simulink model "case2"  (R2024b)
settings: Solver=FixedStepAuto  StartTime=0  StopTime=1  FixedStep=1e-7  RelTol=1e-3
values from neighbouring files (symbols this model uses):
  SG_D_1_D = 0.01056    [IEEE9_case_parameters.m]    (also in case1_parameters.m; case2_parameters.m; case3_parameters.m; case4_parameters.m)
  SG_D_1_EnableSaturation = 0    [IEEE9_case_parameters.m]    (also in case1_parameters.m; case2_parameters.m; case3_parameters.m; case4_parameters.m)
  SG_D_1_f0 = 60    [IEEE9_case_parameters.m]    (also in case1_parameters.m; case2_parameters.m; case3_parameters.m; case4_parameters.m)
  SG_D_1_H = 7.5    [IEEE9_case_parameters.m]    (also in case1_parameters.m; case2_parameters.m; case3_parameters.m; case4_parameters.m)
  SG_D_1_K_A = 20    [IEEE9_case_parameters.m]    (also in case1_parameters.m; case2_parameters.m; case3_parameters.m; case4_parameters.m)
  SG_D_1_K_E = 1.000000e+1    (= 10)    [IEEE9_case_parameters.m]    (also in case1_parameters.m; case2_parameters.m; case3_parameters.m; case4_parameters.m)
  SG_D_1_K_F = 2.363    [IEEE9_case_parameters.m]    (also in case1_parameters.m; case2_parameters.m; case3_parameters.m; case4_parameters.m)
  SG_D_1_K_s = 0.5    [IEEE9_case_parameters.m]    (also in case1_parameters.m = 5; case2_parameters.m = 5; case3_parameters.m = 5; case4_parameters.m = 5)
  SG_D_1_R_a = 0.001088    [IEEE9_case_parameters.m]    (also in case1_parameters.m; case2_parameters.m; case3_parameters.m; case4_parameters.m)
  SG_D_1_S_A = 1    [IEEE9_case_parameters.m]    (also in case1_parameters.m; case2_parameters.m; case3_parameters.m; case4_parameters.m)
  SG_D_1_S_B = 0.103    [IEEE9_case_parameters.m]    (also in case1_parameters.m; case2_parameters.m; case3_parameters.m; case4_parameters.m)
  SG_D_1_S_N = 10.659857    [IEEE9_case_parameters.m]    (also in case1_parameters.m; case2_parameters.m; case3_parameters.m; case4_parameters.m)
  SG_D_1_SpeedPara = 200    [IEEE9_case_parameters.m]    (also in case1_parameters.m; case2_parameters.m; case3_parameters.m; case4_parameters.m)
  SG_D_1_T_0 = 0.720173    [IEEE9_case_parameters.m]    (also in case1_parameters.m = 0.755522; case2_parameters.m = 0.808931; case3_parameters.m = 0.869402; case4_parameters.m = 0.729316)
  SG_D_1_T_1 = 0.3    [IEEE9_case_parameters.m]    (also in case1_parameters.m; case2_parameters.m; case3_parameters.m; case4_parameters.m)
  SG_D_1_T_2 = 0.05    [IEEE9_case_parameters.m]    (also in case1_parameters.m; case2_parameters.m; case3_parameters.m; case4_parameters.m)
  SG_D_1_T_3 = 0.02    [IEEE9_case_parameters.m]    (also in case1_parameters.m; case2_parameters.m; case3_parameters.m; case4_parameters.m)
  SG_D_1_T_4 = 0.005    [IEEE9_case_parameters.m]    (also in case1_parameters.m; case2_parameters.m; case3_parameters.m; case4_parameters.m)
  SG_D_1_T_A = 0.02    [IEEE9_case_parameters.m]    (also in case1_parameters.m; case2_parameters.m; case3_parameters.m; case4_parameters.m)
  SG_D_1_T_dd = 8.000000e+0    (= 8)    [IEEE9_case_parameters.m]    (also in case1_parameters.m; case2_parameters.m; case3_parameters.m; case4_parameters.m)
  SG_D_1_T_ddd = 0.04    [IEEE9_case_parameters.m]    (also in case1_parameters.m; case2_parameters.m; case3_parameters.m; case4_parameters.m)
  SG_D_1_T_E = 0.314    [IEEE9_case_parameters.m]    (also in case1_parameters.m; case2_parameters.m; case3_parameters.m; case4_parameters.m)
  SG_D_1_T_F = 0.35    [IEEE9_case_parameters.m]    (also in case1_parameters.m; case2_parameters.m; case3_parameters.m; case4_parameters.m)
  SG_D_1_T_qd = 0.8    [IEEE9_case_parameters.m]    (also in case1_parameters.m; case2_parameters.m; case3_parameters.m; case4_parameters.m)
  SG_D_1_T_qdd = 0.02    [IEEE9_case_parameters.m]    (also in case1_parameters.m; case2_parameters.m; case3_parameters.m; case4_parameters.m)
  SG_D_1_T_speed = 0.1    [IEEE9_case_parameters.m]    (also in case1_parameters.m = 200; case2_parameters.m = 200; case3_parameters.m = 200; case4_parameters.m = 200)
  SG_D_1_T_w = 0.5    [IEEE9_case_parameters.m]    (also in case1_parameters.m; case2_parameters.m; case3_parameters.m; case4_parameters.m)
  SG_D_1_V_ref = 1.990276    [IEEE9_case_parameters.m]    (also in case1_parameters.m = 2.042296; case2_parameters.m = 2.051388; case3_parameters.m = 2.089584; case4_parameters.m = 2.01845)
  SG_D_1_w_ref = 376.991118    [IEEE9_case_parameters.m]    (also in case1_parameters.m; case2_parameters.m; case3_parameters.m; case4_parameters.m)
  SG_D_1_wb = 6.000000e+1    (= 60)    [IEEE9_case_parameters.m]    (also in case1_parameters.m; case2_parameters.m; case3_parameters.m; case4_parameters.m)
  SG_D_1_x_d = 1.9    [IEEE9_case_parameters.m]    (also in case1_parameters.m; case2_parameters.m; case3_parameters.m; case4_parameters.m)
  SG_D_1_x_dd = 0.302    [IEEE9_case_parameters.m]    (also in case1_parameters.m; case2_parameters.m; case3_parameters.m; case4_parameters.m)
  SG_D_1_x_ddd = 0.204    [IEEE9_case_parameters.m]    (also in case1_parameters.m; case2_parameters.m; case3_parameters.m; case4_parameters.m)
  SG_D_1_x_l = 0.05    [IEEE9_case_parameters.m]    (also in case1_parameters.m; case2_parameters.m; case3_parameters.m; case4_parameters.m)
  SG_D_1_x_q = 1.3    [IEEE9_case_parameters.m]    (also in case1_parameters.m; case2_parameters.m; case3_parameters.m; case4_parameters.m)
  SG_D_1_x_qd = 0.5    [IEEE9_case_parameters.m]    (also in case1_parameters.m; case2_parameters.m; case3_parameters.m; case4_parameters.m)
  SG_D_1_x_qdd = 0.3    [IEEE9_case_parameters.m]    (also in case1_parameters.m; case2_parameters.m; case3_parameters.m; case4_parameters.m)
  SG_D_2_D = 0.02    [IEEE9_case_parameters.m]    (also in case1_parameters.m; case2_parameters.m; case3_parameters.m; case4_parameters.m)
  SG_D_2_EnableSaturation = 0    [IEEE9_case_parameters.m]    (also in case1_parameters.m; case2_parameters.m; case3_parameters.m; case4_parameters.m)
  SG_D_2_f0 = 60    [IEEE9_case_parameters.m]    (also in case1_parameters.m; case2_parameters.m; case3_parameters.m; case4_parameters.m)
  SG_D_2_H = 8.000000e+0    (= 8)    [IEEE9_case_parameters.m]    (also in case1_parameters.m; case2_parameters.m; case3_parameters.m; case4_parameters.m)
  SG_D_2_K_A = 20    [IEEE9_case_parameters.m]    (also in case1_parameters.m; case2_parameters.m; case3_parameters.m; case4_parameters.m)
  SG_D_2_K_E = 1.000000e+1    (= 10)    [IEEE9_case_parameters.m]    (also in case1_parameters.m; case2_parameters.m; case3_parameters.m; case4_parameters.m)
  SG_D_2_K_F = 2.363    [IEEE9_case_parameters.m]    (also in case1_parameters.m; case2_parameters.m; case3_parameters.m; case4_parameters.m)
  SG_D_2_K_s = 0.5    [IEEE9_case_parameters.m]    (also in case1_parameters.m = 4; case2_parameters.m = 4; case3_parameters.m = 4; case4_parameters.m = 4)
  SG_D_2_R_a = 0.001088    [IEEE9_case_parameters.m]    (also in case1_parameters.m; case2_parameters.m; case3_parameters.m; case4_parameters.m)
  SG_D_2_S_A = 1    [IEEE9_case_parameters.m]    (also in case1_parameters.m; case2_parameters.m; case3_parameters.m; case4_parameters.m)
  SG_D_2_S_B = 0.103    [IEEE9_case_parameters.m]    (also in case1_parameters.m; case2_parameters.m; case3_parameters.m; case4_parameters.m)
  SG_D_2_S_N = 10.659857    [IEEE9_case_parameters.m]    (also in case1_parameters.m; case2_parameters.m; case3_parameters.m; case4_parameters.m)
  SG_D_2_SpeedPara = 200    [IEEE9_case_parameters.m]    (also in case1_parameters.m; case2_parameters.m; case3_parameters.m; case4_parameters.m)
  SG_D_2_T_0 = 1.632913    [IEEE9_case_parameters.m]    (also in case1_parameters.m = 1.632925; case2_parameters.m = 1.632915; case3_parameters.m = 1.632914; case4_parameters.m = 1.632927)
  SG_D_2_T_1 = 0.2    [IEEE9_case_parameters.m]    (also in case1_parameters.m; case2_parameters.m; case3_parameters.m; case4_parameters.m)
  SG_D_2_T_2 = 0.05    [IEEE9_case_parameters.m]    (also in case1_parameters.m; case2_parameters.m; case3_parameters.m; case4_parameters.m)
  SG_D_2_T_3 = 0.02    [IEEE9_case_parameters.m]    (also in case1_parameters.m; case2_parameters.m; case3_parameters.m; case4_parameters.m)
  SG_D_2_T_4 = 0.005    [IEEE9_case_parameters.m]    (also in case1_parameters.m; case2_parameters.m; case3_parameters.m; case4_parameters.m)
  SG_D_2_T_A = 0.02    [IEEE9_case_parameters.m]    (also in case1_parameters.m; case2_parameters.m; case3_parameters.m; case4_parameters.m)
  SG_D_2_T_dd = 7.9    [IEEE9_case_parameters.m]    (also in case1_parameters.m; case2_parameters.m; case3_parameters.m; case4_parameters.m)
  SG_D_2_T_ddd = 0.04    [IEEE9_case_parameters.m]    (also in case1_parameters.m; case2_parameters.m; case3_parameters.m; case4_parameters.m)
  SG_D_2_T_E = 0.314    [IEEE9_case_parameters.m]    (also in case1_parameters.m; case2_parameters.m; case3_parameters.m; case4_parameters.m)
  SG_D_2_T_F = 0.35    [IEEE9_case_parameters.m]    (also in case1_parameters.m; case2_parameters.m; case3_parameters.m; case4_parameters.m)
  SG_D_2_T_qd = 0.8    [IEEE9_case_parameters.m]    (also in case1_parameters.m; case2_parameters.m; case3_parameters.m; case4_parameters.m)
  SG_D_2_T_qdd = 0.015    [IEEE9_case_parameters.m]    (also in case1_parameters.m; case2_parameters.m; case3_parameters.m; case4_parameters.m)
  SG_D_2_T_speed = 0.1    [IEEE9_case_parameters.m]    (also in case1_parameters.m = 150; case2_parameters.m = 150; case3_parameters.m = 150; case4_parameters.m = 150)
  SG_D_2_T_w = 0.35    [IEEE9_case_parameters.m]    (also in case1_parameters.m; case2_parameters.m; case3_parameters.m; case4_parameters.m)
  SG_D_2_V_ref = 2.58547    [IEEE9_case_parameters.m]    (also in case1_parameters.m = 2.597896; case2_parameters.m = 2.587136; case3_parameters.m = 2.586042; case4_parameters.m = 2.599679)
  SG_D_2_w_ref = 376.991118    [IEEE9_case_parameters.m]    (also in case1_parameters.m; case2_parameters.m; case3_parameters.m; case4_parameters.m)
  SG_D_2_wb = 6.000000e+1    (= 60)    [IEEE9_case_parameters.m]    (also in case1_parameters.m; case2_parameters.m; case3_parameters.m; case4_parameters.m)
  SG_D_2_x_d = 1.8    [IEEE9_case_parameters.m]    (also in case1_parameters.m; case2_parameters.m; case3_parameters.m; case4_parameters.m)
  SG_D_2_x_dd = 0.302    [IEEE9_case_parameters.m]    (also in case1_parameters.m; case2_parameters.m; case3_parameters.m; case4_parameters.m)
  SG_D_2_x_ddd = 0.204    [IEEE9_case_parameters.m]    (also in case1_parameters.m; case2_parameters.m; case3_parameters.m; case4_parameters.m)
  SG_D_2_x_l = 0.05    [IEEE9_case_parameters.m]    (also in case1_parameters.m; case2_parameters.m; case3_parameters.m; case4_parameters.m)
  SG_D_2_x_q = 1.25    [IEEE9_case_parameters.m]    (also in case1_parameters.m; case2_parameters.m; case3_parameters.m; case4_parameters.m)
  SG_D_2_x_qd = 0.5    [IEEE9_case_parameters.m]    (also in case1_parameters.m; case2_parameters.m; case3_parameters.m; case4_parameters.m)
  SG_D_2_x_qdd = 0.3    [IEEE9_case_parameters.m]    (also in case1_parameters.m; case2_parameters.m; case3_parameters.m; case4_parameters.m)
  SG_D_3_D = 0.02    [IEEE9_case_parameters.m]    (also in case1_parameters.m; case2_parameters.m; case3_parameters.m; case4_parameters.m)
  SG_D_3_EnableSaturation = 0    [IEEE9_case_parameters.m]    (also in case1_parameters.m; case2_parameters.m; case3_parameters.m; case4_parameters.m)
  SG_D_3_f0 = 60    [IEEE9_case_parameters.m]    (also in case1_parameters.m; case2_parameters.m; case3_parameters.m; case4_parameters.m)
  SG_D_3_H = 7.7    [IEEE9_case_parameters.m]    (also in case1_parameters.m; case2_parameters.m; case3_parameters.m; case4_parameters.m)
  SG_D_3_K_A = 20    [IEEE9_case_parameters.m]    (also in case1_parameters.m; case2_parameters.m; case3_parameters.m; case4_parameters.m)
  SG_D_3_K_E = 1.000000e+1    (= 10)    [IEEE9_case_parameters.m]    (also in case1_parameters.m; case2_parameters.m; case3_parameters.m; case4_parameters.m)
  SG_D_3_K_F = 2.363    [IEEE9_case_parameters.m]    (also in case1_parameters.m; case2_parameters.m; case3_parameters.m; case4_parameters.m)
  SG_D_3_K_s = 0.2    [IEEE9_case_parameters.m]    (also in case1_parameters.m = 2; case2_parameters.m = 2; case3_parameters.m = 2; case4_parameters.m = 2)
  SG_D_3_R_a = 0.001088    [IEEE9_case_parameters.m]    (also in case1_parameters.m; case2_parameters.m; case3_parameters.m; case4_parameters.m)
  SG_D_3_S_A = 1    [IEEE9_case_parameters.m]    (also in case1_parameters.m; case2_parameters.m; case3_parameters.m; case4_parameters.m)
  SG_D_3_S_B = 0.103    [IEEE9_case_parameters.m]    (also in case1_parameters.m; case2_parameters.m; case3_parameters.m; case4_parameters.m)
  SG_D_3_S_N = 10.659857    [IEEE9_case_parameters.m]    (also in case1_parameters.m; case2_parameters.m; case3_parameters.m; case4_parameters.m)
  SG_D_3_SpeedPara = 200    [IEEE9_case_parameters.m]    (also in case1_parameters.m; case2_parameters.m; case3_parameters.m; case4_parameters.m)
  SG_D_3_T_0 = 0.850788    [IEEE9_case_parameters.m]    (also in case1_parameters.m = 0.850786; case2_parameters.m = 0.850787; case3_parameters.m; case4_parameters.m = 0.850786)
  SG_D_3_T_1 = 0.2    [IEEE9_case_parameters.m]    (also in case1_parameters.m; case2_parameters.m; case3_parameters.m; case4_parameters.m)
  SG_D_3_T_2 = 0.05    [IEEE9_case_parameters.m]    (also in case1_parameters.m; case2_parameters.m; case3_parameters.m; case4_parameters.m)
  SG_D_3_T_3 = 0.02    [IEEE9_case_parameters.m]    (also in case1_parameters.m; case2_parameters.m; case3_parameters.m; case4_parameters.m)
  SG_D_3_T_4 = 0.005    [IEEE9_case_parameters.m]    (also in case1_parameters.m; case2_parameters.m; case3_parameters.m; case4_parameters.m)
  SG_D_3_T_A = 0.02    [IEEE9_case_parameters.m]    (also in case1_parameters.m; case2_parameters.m; case3_parameters.m; case4_parameters.m)
  SG_D_3_T_dd = 8.1    [IEEE9_case_parameters.m]    (also in case1_parameters.m; case2_parameters.m; case3_parameters.m; case4_parameters.m)
  SG_D_3_T_ddd = 0.04    [IEEE9_case_parameters.m]    (also in case1_parameters.m; case2_parameters.m; case3_parameters.m; case4_parameters.m)
  SG_D_3_T_E = 0.314    [IEEE9_case_parameters.m]    (also in case1_parameters.m; case2_parameters.m; case3_parameters.m; case4_parameters.m)
  SG_D_3_T_F = 0.35    [IEEE9_case_parameters.m]    (also in case1_parameters.m; case2_parameters.m; case3_parameters.m; case4_parameters.m)
  SG_D_3_T_qd = 0.8    [IEEE9_case_parameters.m]    (also in case1_parameters.m; case2_parameters.m; case3_parameters.m; case4_parameters.m)
  SG_D_3_T_qdd = 0.015    [IEEE9_case_parameters.m]    (also in case1_parameters.m; case2_parameters.m; case3_parameters.m; case4_parameters.m)
  SG_D_3_T_speed = 0.1    [IEEE9_case_parameters.m]    (also in case1_parameters.m = 180; case2_parameters.m = 180; case3_parameters.m = 180; case4_parameters.m = 180)
  SG_D_3_T_w = 0.4    [IEEE9_case_parameters.m]    (also in case1_parameters.m; case2_parameters.m; case3_parameters.m; case4_parameters.m)
  SG_D_3_V_ref = 1.892727    [IEEE9_case_parameters.m]    (also in case1_parameters.m = 1.906439; case2_parameters.m = 1.895535; case3_parameters.m = 1.892105; case4_parameters.m = 1.906598)
  SG_D_3_w_ref = 376.991118    [IEEE9_case_parameters.m]    (also in case1_parameters.m; case2_parameters.m; case3_parameters.m; case4_parameters.m)
  SG_D_3_wb = 6.000000e+1    (= 60)    [IEEE9_case_parameters.m]    (also in case1_parameters.m; case2_parameters.m; case3_parameters.m; case4_parameters.m)
  SG_D_3_x_d = 1.85    [IEEE9_case_parameters.m]    (also in case1_parameters.m; case2_parameters.m; case3_parameters.m; case4_parameters.m)
  SG_D_3_x_dd = 0.302    [IEEE9_case_parameters.m]    (also in case1_parameters.m; case2_parameters.m; case3_parameters.m; case4_parameters.m)
  SG_D_3_x_ddd = 0.204    [IEEE9_case_parameters.m]    (also in case1_parameters.m; case2_parameters.m; case3_parameters.m; case4_parameters.m)
  SG_D_3_x_l = 0.05    [IEEE9_case_parameters.m]    (also in case1_parameters.m; case2_parameters.m; case3_parameters.m; case4_parameters.m)
  SG_D_3_x_q = 1.2    [IEEE9_case_parameters.m]    (also in case1_parameters.m; case2_parameters.m; case3_parameters.m; case4_parameters.m)
  SG_D_3_x_qd = 0.5    [IEEE9_case_parameters.m]    (also in case1_parameters.m; case2_parameters.m; case3_parameters.m; case4_parameters.m)
  SG_D_3_x_qdd = 0.3    [IEEE9_case_parameters.m]    (also in case1_parameters.m; case2_parameters.m; case3_parameters.m; case4_parameters.m)
(part 8 of 12)

== system case2/SG_D_2/d_psi_d_SG_D_2_block ==
  note: d_psi_d_SG_D_2 in case2
      | $2\,\pi \,f_{0}\,\left(v_{d,\mathrm{SG},D,2}\,\sin\left(\theta _{\mathrm{SG},D,2}\right)-v_{q,\mathrm{SG},D,2}\,\cos\left(\theta _{\mathrm{SG},D,2}\right)+\frac{R_{a}\,\left(\frac{\psi _{\mathrm{1d},\mathrm{SG},D,2}\,\left(x_{\mathrm{dd}}-x_{\mathrm{ddd}}\right)}{x_{\mathrm{dd}}-x_{l}}-\psi _{d,\mathrm{SG},D,2}+\frac{\psi _{\mathrm{fd},\mathrm{SG},D,2}\,\left(x_{\mathrm{ddd}}-x_{l}\right)}{x_{\mathrm{dd}}-x_{l}}\right)}{x_{\mathrm{ddd}}}+\frac{\psi _{q,\mathrm{SG},D,2}\,w_{\mathrm{SG},D,2}}{2\,f_{0}\,\pi }\right)$
      | Automatically generated on 2025-10-31 18:54:12 .
  State_psi_1d_SG_D_2_3fdee : Inport
  State_psi_d_SG_D_2_d60ed : Inport  Port=2
  State_psi_fd_SG_D_2_19126 : Inport  Port=3
  Input_v_d_SG_D_2_3ae72 : Inport  Port=4
  State_theta_SG_D_2_01400 : Inport  Port=5
  Input_v_q_SG_D_2_cabf7 : Inport  Port=6
  State_theta_SG_D_2_a0973 : Inport  Port=7
  State_psi_q_SG_D_2_fe7e7 : Inport  Port=8
  State_w_SG_D_2_e892d : Inport  Port=9
  Add_2c66e : Sum
  Add_408a3 : Sum
  Constant_-1_07947 : Constant  Value=-1
  Constant_-2.0_4d0c8 : Constant  Value=-2.0
  Constant_2.0_2af4c : Constant  Value=2.0
  Constant_R_a_dbd06 : Constant  Value=R_a
  Constant_f0_83e57 : Constant  Value=f0
  Constant_f0_9e5d9 : Constant  Value=f0
  Constant_pi_c86ee : Constant  Value=pi
  Constant_pi_d09dc : Constant  Value=pi
  Constant_x_dd_68bb8 : Constant  Value=x_dd
  Constant_x_dd_73140 : Constant  Value=x_dd
  Constant_x_dd_7f225 : Constant  Value=x_dd
  Constant_x_ddd_754dc : Constant  Value=x_ddd
  Constant_x_ddd_c9197 : Constant  Value=x_ddd
  Constant_x_ddd_e8b22 : Constant  Value=x_ddd
  Constant_x_l_4c35a : Constant  Value=x_l
  Constant_x_l_e9676 : Constant  Value=x_l
  Constant_x_l_f0ba1 : Constant  Value=x_l
  Divide_25f7b : Product  Inputs=*/
  Divide_6b17e : Product  Inputs=*/
  Divide_7e72f : Product  Inputs=*/
  Divide_aeaf3 : Product  Inputs=*/
  MathFunc_cos_20e10 : Trigonometry  Operator=cos
  MathFunc_sin_874eb : Trigonometry
  Product_12c06 : Product
  Product_1e44e : Product
  Product_2ec50 : Product
  Product_4577d : Product
  Product_4597d : Product
  Product_52fae : Product
  Product_61ff6 : Product
  Product_88970 : Product
  Product_92e21 : Product
  Product_9afb2 : Product
  Product_9ba31 : Product
  Product_c6f43 : Product
  Subtract_063f9 : Sum  Inputs=+-
  Subtract_351ed : Sum  Inputs=+-
  Subtract_90ebb : Sum  Inputs=+-
  Subtract_bd665 : Sum  Inputs=+-
  Subtract_bec5b : Sum  Inputs=+-
  Subtract_c952b : Sum  Inputs=+-
  Subtract_fa91f : Sum  Inputs=+-
  Blockout_d_psi_d_SG_D_2_b24b5 : Outport
  wires:
  MathFunc_sin_874eb/1 -> Product_4597d/2
  Constant_x_dd_73140/1 -> Subtract_063f9/1
  Constant_-1_07947/1 -> Product_9ba31/1
  Constant_x_l_f0ba1/1 -> Subtract_063f9/2
  State_psi_1d_SG_D_2_3fdee/1 -> Product_9ba31/2
  Constant_f0_9e5d9/1 -> Product_52fae/2
  Constant_2.0_2af4c/1 -> Product_1e44e/1
  Constant_x_l_e9676/1 -> Subtract_351ed/2
  Constant_x_dd_68bb8/1 -> Subtract_bd665/1
  Product_9afb2/1 -> Blockout_d_psi_d_SG_D_2_b24b5/1
  Constant_pi_c86ee/1 -> Product_1e44e/2
  Constant_x_ddd_e8b22/1 -> Subtract_bd665/2
  Subtract_bec5b/1 -> Product_9afb2/2
  Product_9ba31/1 -> Product_61ff6/1
  Product_1e44e/1 -> Product_4577d/1
  Subtract_bd665/1 -> Product_61ff6/2
  Divide_aeaf3/1 -> Subtract_bec5b/2
  Constant_x_ddd_754dc/1 -> Subtract_c952b/1
  Constant_x_l_4c35a/1 -> Subtract_c952b/2
  Product_61ff6/1 -> Divide_6b17e/1
  Subtract_90ebb/1 -> Add_408a3/1
  Subtract_063f9/1 -> Divide_6b17e/2
  State_psi_fd_SG_D_2_19126/1 -> Product_2ec50/1
  Subtract_c952b/1 -> Product_2ec50/2
  Constant_x_dd_7f225/1 -> Subtract_351ed/1
  Divide_6b17e/1 -> Add_2c66e/1
  State_psi_d_SG_D_2_d60ed/1 -> Add_2c66e/2
  Product_2ec50/1 -> Divide_25f7b/1
  Subtract_351ed/1 -> Divide_25f7b/2
  Add_2c66e/1 -> Subtract_fa91f/1
  Divide_25f7b/1 -> Subtract_fa91f/2
  Constant_R_a_dbd06/1 -> Product_88970/1
  Subtract_fa91f/1 -> Product_88970/2
  Divide_7e72f/1 -> Subtract_90ebb/1
  State_theta_SG_D_2_01400/1 -> MathFunc_sin_874eb/1
  Product_88970/1 -> Divide_7e72f/1
  Constant_-2.0_4d0c8/1 -> Product_92e21/1
  Input_v_d_SG_D_2_3ae72/1 -> Product_4597d/1
  Constant_x_ddd_c9197/1 -> Divide_7e72f/2
  State_theta_SG_D_2_a0973/1 -> MathFunc_cos_20e10/1
  Product_52fae/1 -> Product_9afb2/1
  Product_4597d/1 -> Subtract_90ebb/2
  Product_92e21/1 -> Product_52fae/1
  Input_v_q_SG_D_2_cabf7/1 -> Product_c6f43/1
  MathFunc_cos_20e10/1 -> Product_c6f43/2
  State_psi_q_SG_D_2_fe7e7/1 -> Product_12c06/1
  State_w_SG_D_2_e892d/1 -> Product_12c06/2
  Constant_f0_83e57/1 -> Product_4577d/2
  Constant_pi_d09dc/1 -> Product_92e21/2
  Product_c6f43/1 -> Add_408a3/2
  Product_12c06/1 -> Divide_aeaf3/1
  Product_4577d/1 -> Divide_aeaf3/2
  Add_408a3/1 -> Subtract_bec5b/1

== system case2/SG_D_2/d_psi_fd_SG_D_2_block ==
  note: d_psi_fd_SG_D_2 in case2
      | $-\frac{\psi _{\mathrm{fd},\mathrm{SG},D,2}-E_{\mathrm{fd},\mathrm{SG},D,2}+\left(x_{d}-x_{\mathrm{dd}}\right)\,\left(\frac{\frac{\psi _{\mathrm{1d},\mathrm{SG},D,2}\,\left(x_{\mathrm{dd}}-x_{\mathrm{ddd}}\right)}{x_{\mathrm{dd}}-x_{l}}-\psi _{d,\mathrm{SG},D,2}+\frac{\psi _{\mathrm{fd},\mathrm{SG},D,2}\,\left(x_{\mathrm{ddd}}-x_{l}\right)}{x_{\mathrm{dd}}-x_{l}}}{x_{\mathrm{ddd}}}-\frac{\left(x_{\mathrm{dd}}-x_{\mathrm{ddd}}\right)\,\left(\psi _{\mathrm{1d},\mathrm{SG},D,2}-\psi _{\mathrm{fd},\mathrm{SG},D,2}+\frac{\left(x_{\mathrm{dd}}-x_{l}\right)\,\left(\frac{\psi _{\mathrm{1d},\mathrm{SG},D,2}\,\left(x_{\mathrm{dd}}-x_{\mathrm{ddd}}\right)}{x_{\mathrm{dd}}-x_{l}}-\psi _{d,\mathrm{SG},D,2}+\frac{\psi _{\mathrm{fd},\mathrm{SG},D,2}\,\left(x_{\mathrm{ddd}}-x_{l}\right)}{x_{\mathrm{dd}}-x_{l}}\right)}{x_{\mathrm{ddd}}}\right)}{{\left(x_{\mathrm{dd}}-x_{l}\right)}^2}\right)}{T_{\mathrm{dd}}}$
      | Automatically generated on 2025-10-31 18:54:21 .
  State_E_fd_SG_D_2_538cb : Inport
  State_psi_fd_SG_D_2_9a5f7 : Inport  Port=2
  State_psi_1d_SG_D_2_9e249 : Inport  Port=3
  State_psi_fd_SG_D_2_7d5d1 : Inport  Port=4
  State_psi_1d_SG_D_2_19e55 : Inport  Port=5
  State_psi_d_SG_D_2_bc679 : Inport  Port=6
  State_psi_fd_SG_D_2_aa5d6 : Inport  Port=7
  State_psi_1d_SG_D_2_c9b22 : Inport  Port=8
  State_psi_d_SG_D_2_749a1 : Inport  Port=9
  State_psi_fd_SG_D_2_e8112 : Inport  Port=10
  Add_45e73 : Sum
  Add_58c29 : Sum
  Constant_-1_cf4fd : Constant  Value=-1
  Constant_-1_d8bec : Constant  Value=-1
  Constant_-1_f602a : Constant  Value=-1
  Constant_2.0_d041e : Constant  Value=2.0
  Constant_T_dd_cb9b1 : Constant  Value=T_dd
  Constant_x_d_60901 : Constant  Value=x_d
  Constant_x_dd_093be : Constant  Value=x_dd
  Constant_x_dd_1490c : Constant  Value=x_dd
  Constant_x_dd_4fc03 : Constant  Value=x_dd
  Constant_x_dd_79bd8 : Constant  Value=x_dd
  Constant_x_dd_7d8ae : Constant  Value=x_dd
  Constant_x_dd_7ef3a : Constant  Value=x_dd
  Constant_x_dd_9b0b0 : Constant  Value=x_dd
  Constant_x_dd_aaa44 : Constant  Value=x_dd
  Constant_x_dd_f4b2d : Constant  Value=x_dd
  Constant_x_dd_fdbea : Constant  Value=x_dd
  Constant_x_ddd_298fe : Constant  Value=x_ddd
  Constant_x_ddd_437aa : Constant  Value=x_ddd
  Constant_x_ddd_4535d : Constant  Value=x_ddd
  Constant_x_ddd_50f36 : Constant  Value=x_ddd
  Constant_x_ddd_bfea8 : Constant  Value=x_ddd
  Constant_x_ddd_c1140 : Constant  Value=x_ddd
  Constant_x_ddd_d07bc : Constant  Value=x_ddd
  Constant_x_l_13584 : Constant  Value=x_l
  Constant_x_l_1b585 : Constant  Value=x_l
  Constant_x_l_5d924 : Constant  Value=x_l
  Constant_x_l_62863 : Constant  Value=x_l
  Constant_x_l_94f7d : Constant  Value=x_l
  Constant_x_l_99b34 : Constant  Value=x_l
  Constant_x_l_cca13 : Constant  Value=x_l
  Constant_x_l_df858 : Constant  Value=x_l
  Divide_09bd1 : Product  Inputs=*/
  Divide_15ee7 : Product  Inputs=*/
  Divide_272be : Product  Inputs=*/
  Divide_49270 : Product  Inputs=*/
  Divide_4ceeb : Product  Inputs=*/
  Divide_62133 : Product  Inputs=*/
  Divide_9829c : Product  Inputs=*/
  Divide_c085e : Product  Inputs=*/
  Power_95e32 : Math  Operator=pow
  Product_25e68 : Product
  Product_2c785 : Product
  Product_31ca3 : Product
  Product_3cb2e : Product
  Product_8bfc0 : Product
  Product_8f3c5 : Product
  Product_9007c : Product
  Product_cbcdb : Product
  Product_d4e32 : Product
  Product_da1d1 : Product
  Subtract_05c6c : Sum  Inputs=+-
  Subtract_0ae45 : Sum  Inputs=+-
  Subtract_11c1b : Sum  Inputs=+-
  Subtract_1448b : Sum  Inputs=+-
  Subtract_1c391 : Sum  Inputs=+-
  Subtract_1c983 : Sum  Inputs=+-
  Subtract_2a91d : Sum  Inputs=+-
  Subtract_402bf : Sum  Inputs=+-
  Subtract_4e5a4 : Sum  Inputs=+-
  Subtract_516c7 : Sum  Inputs=+-
  Subtract_6f371 : Sum  Inputs=+-
  Subtract_79704 : Sum  Inputs=+-
  Subtract_967be : Sum  Inputs=+-
  Subtract_a2f53 : Sum  Inputs=+-
  Subtract_a7caa : Sum  Inputs=+-
  Subtract_cdc47 : Sum  Inputs=+-
  Subtract_e24f1 : Sum  Inputs=+-
  Subtract_ebde2 : Sum  Inputs=+-
  Subtract_eccf3 : Sum  Inputs=+-
  Blockout_d_psi_fd_SG_D_2_3c09c : Outport
  wires:
  Constant_x_dd_79bd8/1 -> Subtract_05c6c/1
  Constant_-1_cf4fd/1 -> Product_2c785/1
  Constant_x_l_99b34/1 -> Subtract_e24f1/2
  Divide_15ee7/1 -> Add_45e73/1
  Subtract_967be/1 -> Product_d4e32/2
  Constant_x_l_1b585/1 -> Subtract_05c6c/2
  Product_d4e32/1 -> Divide_9829c/1
  State_psi_1d_SG_D_2_19e55/1 -> Product_2c785/2
  Constant_x_dd_4fc03/1 -> Subtract_516c7/1
  Product_3cb2e/1 -> Divide_15ee7/1
  Constant_x_dd_1490c/1 -> Subtract_1448b/1
  Constant_x_ddd_4535d/1 -> Subtract_516c7/2
  Constant_x_dd_7d8ae/1 -> Subtract_1c983/1
  Product_2c785/1 -> Product_cbcdb/1
  Subtract_516c7/1 -> Product_cbcdb/2
  State_psi_d_SG_D_2_749a1/1 -> Add_45e73/2
  Constant_x_ddd_298fe/1 -> Subtract_967be/1
  Constant_x_l_62863/1 -> Subtract_967be/2
  Product_cbcdb/1 -> Divide_4ceeb/1
  Subtract_05c6c/1 -> Divide_4ceeb/2
  State_psi_fd_SG_D_2_aa5d6/1 -> Product_d4e32/1
  Subtract_ebde2/1 -> Product_9007c/2
  Constant_x_dd_093be/1 -> Subtract_0ae45/1
  Constant_x_l_13584/1 -> Subtract_0ae45/2
  Product_8bfc0/1 -> Product_9007c/1
  Divide_4ceeb/1 -> Add_58c29/1
  State_psi_d_SG_D_2_bc679/1 -> Add_58c29/2
  Subtract_0ae45/1 -> Divide_9829c/2
  Constant_x_dd_aaa44/1 -> Subtract_e24f1/1
  Constant_x_ddd_437aa/1 -> Subtract_11c1b/1
  Add_58c29/1 -> Subtract_402bf/1
  Divide_9829c/1 -> Subtract_402bf/2
  Constant_-1_f602a/1 -> Product_8f3c5/1
  Product_25e68/1 -> Divide_c085e/1
  State_psi_1d_SG_D_2_c9b22/1 -> Product_8f3c5/2
  Subtract_1448b/1 -> Product_8bfc0/2
  Constant_x_dd_9b0b0/1 -> Subtract_cdc47/1
  Divide_c085e/1 -> Subtract_6f371/2
  Constant_-1_d8bec/1 -> Product_8bfc0/1
  Constant_x_ddd_d07bc/1 -> Subtract_cdc47/2
  Constant_x_ddd_50f36/1 -> Divide_272be/2
  Subtract_e24f1/1 -> Product_da1d1/1
  Subtract_402bf/1 -> Product_da1d1/2
  State_psi_fd_SG_D_2_7d5d1/1 -> Subtract_eccf3/2
  Product_8f3c5/1 -> Product_3cb2e/1
  Subtract_cdc47/1 -> Product_3cb2e/2
  Constant_2.0_d041e/1 -> Power_95e32/2
  State_psi_1d_SG_D_2_9e249/1 -> Subtract_eccf3/1
  Constant_x_dd_f4b2d/1 -> Subtract_1c391/1
  Subtract_11c1b/1 -> Product_25e68/2
  Constant_x_l_94f7d/1 -> Subtract_1c391/2
  Constant_x_l_5d924/1 -> Subtract_11c1b/2
  Constant_x_ddd_bfea8/1 -> Subtract_1448b/2
  Subtract_1c983/1 -> Divide_c085e/2
  Product_da1d1/1 -> Divide_272be/1
  Subtract_1c391/1 -> Divide_15ee7/2
  State_psi_fd_SG_D_2_e8112/1 -> Product_25e68/1
  Constant_x_l_cca13/1 -> Subtract_1c983/2
  Constant_x_dd_7ef3a/1 -> Subtract_a2f53/1
  Subtract_eccf3/1 -> Subtract_ebde2/1
  Divide_272be/1 -> Subtract_ebde2/2
  Constant_x_l_df858/1 -> Subtract_a2f53/2
  Subtract_a2f53/1 -> Power_95e32/1
  Add_45e73/1 -> Subtract_6f371/1
  Product_9007c/1 -> Divide_09bd1/1
  Power_95e32/1 -> Divide_09bd1/2
  Subtract_6f371/1 -> Divide_62133/1
  Constant_x_ddd_c1140/1 -> Divide_62133/2
  Constant_x_d_60901/1 -> Subtract_2a91d/1
  Constant_x_dd_fdbea/1 -> Subtract_2a91d/2
  Divide_09bd1/1 -> Subtract_a7caa/1
  Divide_62133/1 -> Subtract_a7caa/2
  State_E_fd_SG_D_2_538cb/1 -> Subtract_4e5a4/1
  State_psi_fd_SG_D_2_9a5f7/1 -> Subtract_4e5a4/2
  Subtract_2a91d/1 -> Product_31ca3/1
  Subtract_a7caa/1 -> Product_31ca3/2
  Subtract_4e5a4/1 -> Subtract_79704/1
  Product_31ca3/1 -> Subtract_79704/2
  Subtract_79704/1 -> Divide_49270/1
  Constant_T_dd_cb9b1/1 -> Divide_49270/2
  Divide_49270/1 -> Blockout_d_psi_fd_SG_D_2_3c09c/1

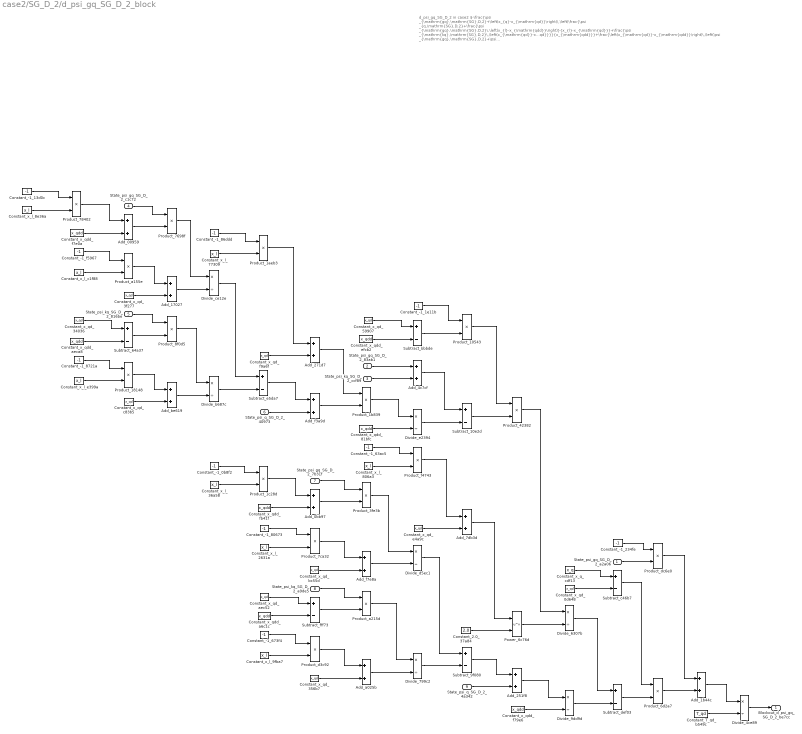
== system case2/SG_D_2/d_psi_gq_SG_D_2_block ==
  note: d_psi_gq_SG_D_2 in case2
      | $-\frac{\psi _{\mathrm{gq},\mathrm{SG},D,2}+\left(x_{q}-x_{\mathrm{qd}}\right)\,\left(\frac{\psi _{q,\mathrm{SG},D,2}+\frac{\psi _{\mathrm{gq},\mathrm{SG},D,2}\,\left(x_{l}-x_{\mathrm{qdd}}\right)}{x_{l}-x_{\mathrm{qd}}}+\frac{\psi _{\mathrm{kq},\mathrm{SG},D,2}\,\left(x_{\mathrm{qd}}-x_{\mathrm{qdd}}\right)}{x_{l}-x_{\mathrm{qd}}}}{x_{\mathrm{qdd}}}+\frac{\left(x_{\mathrm{qd}}-x_{\mathrm{qdd}}\right)\,\left(\psi _{\mathrm{gq},\mathrm{SG},D,2}+\psi _{\mathrm{kq},\mathrm{SG},D,2}+\frac{\left(x_{l}-x_{\mathrm{qd}}\right)\,\left(\psi _{q,\mathrm{SG},D,2}+\frac{\psi _{\mathrm{gq},\mathrm{SG},D,2}\,\left(x_{l}-x_{\mathrm{qdd}}\right)}{x_{l}-x_{\mathrm{qd}}}+\frac{\psi _{\mathrm{kq},\mathrm{SG},D,2}\,\left(x_{\mathrm{qd}}-x_{\mathrm{qdd}}\right)}{x_{l}-x_{\mathrm{qd}}}\right)}{x_{\mathrm{qdd}}}\right)}{{\left(x_{l}-x_{\mathrm{qd}}\right)}^2}\right)}{T_{\mathrm{qd}}}$
      | Automatically generated on 2025-10-31 18:54:30 .
  State_psi_gq_SG_D_2_a2a06 : Inport
  State_psi_gq_SG_D_2_83ab1 : Inport  Port=2
  State_psi_kq_SG_D_2_ccf89 : Inport  Port=3
  State_psi_gq_SG_D_2_c1c72 : Inport  Port=4
  State_psi_kq_SG_D_2_816be : Inport  Port=5
  State_psi_q_SG_D_2_40973 : Inport  Port=6
  State_psi_gq_SG_D_2_7b31f : Inport  Port=7
  State_psi_kq_SG_D_2_a9de5 : Inport  Port=8
  State_psi_q_SG_D_2_4a342 : Inport  Port=9
  Add_00959 : Sum
  Add_0bb97 : Sum
  Add_17027 : Sum
  Add_1b44c : Sum
  Add_251f8 : Sum
  Add_271d7 : Sum
  Add_4c7cf : Sum
  Add_7db3d : Sum
  Add_a025b : Sum
  Add_be619 : Sum
  Add_f3a9d : Sum
  Add_f7e8a : Sum
  Constant_-1_0b8f2 : Constant  Value=-1
  Constant_-1_13d0c : Constant  Value=-1
  Constant_-1_1e11b : Constant  Value=-1
  Constant_-1_234fe : Constant  Value=-1
  Constant_-1_63ac5 : Constant  Value=-1
  Constant_-1_673f4 : Constant  Value=-1
  Constant_-1_80673 : Constant  Value=-1
  Constant_-1_86ddd : Constant  Value=-1
  Constant_-1_8721a : Constant  Value=-1
  Constant_-1_f5967 : Constant  Value=-1
  Constant_2.0_37a84 : Constant  Value=2.0
  Constant_T_qd_b549c : Constant  Value=T_qd
  Constant_x_l_2631a : Constant  Value=x_l
  Constant_x_l_36a58 : Constant  Value=x_l
  Constant_x_l_77309 : Constant  Value=x_l
  Constant_x_l_806a3 : Constant  Value=x_l
  Constant_x_l_8e36a : Constant  Value=x_l
  Constant_x_l_9fba7 : Constant  Value=x_l
  Constant_x_l_c1f88 : Constant  Value=x_l
  Constant_x_l_e399a : Constant  Value=x_l
  Constant_x_q_cdf13 : Constant  Value=x_q
  Constant_x_qd_0d648 : Constant  Value=x_qd
  Constant_x_qd_34036 : Constant  Value=x_qd
  Constant_x_qd_356b7 : Constant  Value=x_qd
  Constant_x_qd_3f277 : Constant  Value=x_qd
  Constant_x_qd_59907 : Constant  Value=x_qd
  Constant_x_qd_aec52 : Constant  Value=x_qd
  Constant_x_qd_bc55d : Constant  Value=x_qd
  Constant_x_qd_c83b5 : Constant  Value=x_qd
  Constant_x_qd_e4a9c : Constant  Value=x_qd
  Constant_x_qd_f9a6f : Constant  Value=x_qd
  Constant_x_qdd_81bfc : Constant  Value=x_qdd
  Constant_x_qdd_a6c1c : Constant  Value=x_qdd
  Constant_x_qdd_aeca8 : Constant  Value=x_qdd
  Constant_x_qdd_efcb2 : Constant  Value=x_qdd
  Constant_x_qdd_f79e6 : Constant  Value=x_qdd
  Constant_x_qdd_f7e0a : Constant  Value=x_qdd
  Constant_x_qdd_fb41f : Constant  Value=x_qdd
  Divide_4ce89 : Product  Inputs=*/
  Divide_6307b : Product  Inputs=*/
  Divide_799c2 : Product  Inputs=*/
  Divide_9dd9d : Product  Inputs=*/
  Divide_b687c : Product  Inputs=*/
  Divide_ce12e : Product  Inputs=*/
  Divide_d5ec1 : Product  Inputs=*/
  Divide_e2394 : Product  Inputs=*/
  Power_6c76d : Math  Operator=pow
  Product_{10543,18148,42382,78402} (4 alike) : Product
  Product_1aeb3 : Product
  Product_1b839 : Product
  Product_1c28d : Product
  Product_3fe3b : Product
  Product_6d2a7 : Product
  Product_7698f : Product
  Product_7ca32 : Product
  Product_8f0d5 : Product
  Product_a155e : Product
  Product_a215d : Product
  Product_d3c92 : Product
  Product_dc6e0 : Product
  Product_f4743 : Product
  Subtract_10e2d : Sum  Inputs=+-
  Subtract_64a37 : Sum  Inputs=+-
  Subtract_9f080 : Sum  Inputs=+-
  Subtract_bbbde : Sum  Inputs=+-
  Subtract_c46b7 : Sum  Inputs=+-
  Subtract_def03 : Sum  Inputs=+-
  Subtract_e5da7 : Sum  Inputs=+-
  Subtract_fff73 : Sum  Inputs=+-
  Blockout_d_psi_gq_SG_D_2_be7cc : Outport
  wires:
  Constant_x_l_9fba7/1 -> Product_d3c92/2
  Constant_x_l_36a58/1 -> Product_1c28d/2
  Constant_x_qd_34036/1 -> Subtract_64a37/1
  Constant_x_l_806a3/1 -> Product_f4743/2
  Constant_x_qdd_efcb2/1 -> Subtract_bbbde/2
  Constant_-1_8721a/1 -> Product_18148/1
  Constant_-1_13d0c/1 -> Product_78402/1
  State_psi_gq_SG_D_2_83ab1/1 -> Add_4c7cf/1
  Constant_x_qdd_aeca8/1 -> Subtract_64a37/2
  Constant_x_qd_59907/1 -> Subtract_bbbde/1
  Constant_x_l_e399a/1 -> Product_18148/2
  Constant_x_l_8e36a/1 -> Product_78402/2
  Product_18148/1 -> Add_be619/1
  Product_78402/1 -> Add_00959/1
  Constant_x_l_c1f88/1 -> Product_a155e/2
  Constant_x_l_77309/1 -> Product_1aeb3/2
  Constant_x_qd_c83b5/1 -> Add_be619/2
  Constant_x_qdd_f7e0a/1 -> Add_00959/2
  Constant_-1_f5967/1 -> Product_a155e/1
  Constant_x_qd_356b7/1 -> Add_a025b/2
  Constant_x_qdd_fb41f/1 -> Add_0bb97/2
  State_psi_gq_SG_D_2_c1c72/1 -> Product_7698f/1
  Add_be619/1 -> Divide_b687c/2
  Add_00959/1 -> Product_7698f/2
  Constant_x_qd_0d648/1 -> Subtract_c46b7/2
  Product_a155e/1 -> Add_17027/1
  Constant_x_qd_3f277/1 -> Add_17027/2
  State_psi_kq_SG_D_2_816be/1 -> Product_8f0d5/1
  Divide_ce12e/1 -> Subtract_e5da7/1
  Subtract_64a37/1 -> Product_8f0d5/2
  Product_7698f/1 -> Divide_ce12e/1
  Add_17027/1 -> Divide_ce12e/2
  Add_f3a9d/1 -> Product_1b839/2
  Product_8f0d5/1 -> Divide_b687c/1
  Constant_-1_86ddd/1 -> Product_1aeb3/1
  Divide_b687c/1 -> Subtract_e5da7/2
  Constant_-1_673f4/1 -> Product_d3c92/1
  Constant_-1_0b8f2/1 -> Product_1c28d/1
  Product_1aeb3/1 -> Add_271d7/1
  Constant_x_qdd_a6c1c/1 -> Subtract_fff73/2
  Constant_x_qd_f9a6f/1 -> Add_271d7/2
  Subtract_e5da7/1 -> Add_f3a9d/1
  Constant_-1_63ac5/1 -> Product_f4743/1
  State_psi_q_SG_D_2_40973/1 -> Add_f3a9d/2
  Product_d3c92/1 -> Add_a025b/1
  Product_1c28d/1 -> Add_0bb97/1
  Constant_-1_80673/1 -> Product_7ca32/1
  Product_1b839/1 -> Divide_e2394/1
  Constant_x_l_2631a/1 -> Product_7ca32/2
  Product_6d2a7/1 -> Add_1b44c/2
  Constant_x_qd_aec52/1 -> Subtract_fff73/1
  Add_271d7/1 -> Product_1b839/1
  State_psi_gq_SG_D_2_7b31f/1 -> Product_3fe3b/1
  Add_a025b/1 -> Divide_799c2/2
  Add_0bb97/1 -> Product_3fe3b/2
  Product_7ca32/1 -> Add_f7e8a/1
  Constant_x_qd_bc55d/1 -> Add_f7e8a/2
  State_psi_kq_SG_D_2_a9de5/1 -> Product_a215d/1
  Subtract_fff73/1 -> Product_a215d/2
  Divide_799c2/1 -> Subtract_9f080/2
  State_psi_kq_SG_D_2_ccf89/1 -> Add_4c7cf/2
  Product_a215d/1 -> Divide_799c2/1
  Constant_x_qdd_81bfc/1 -> Divide_e2394/2
  Product_3fe3b/1 -> Divide_d5ec1/1
  Add_f7e8a/1 -> Divide_d5ec1/2
  Constant_-1_1e11b/1 -> Product_10543/1
  Subtract_bbbde/1 -> Product_10543/2
  Add_4c7cf/1 -> Subtract_10e2d/1
  Divide_e2394/1 -> Subtract_10e2d/2
  Product_f4743/1 -> Add_7db3d/1
  Constant_x_qd_e4a9c/1 -> Add_7db3d/2
  Divide_d5ec1/1 -> Subtract_9f080/1
  Product_10543/1 -> Product_42382/1
  Subtract_10e2d/1 -> Product_42382/2
  Add_7db3d/1 -> Power_6c76d/1
  Constant_2.0_37a84/1 -> Power_6c76d/2
  Subtract_9f080/1 -> Add_251f8/1
  State_psi_q_SG_D_2_4a342/1 -> Add_251f8/2
  Product_42382/1 -> Divide_6307b/1
  Power_6c76d/1 -> Divide_6307b/2
  Add_251f8/1 -> Divide_9dd9d/1
  Constant_x_qdd_f79e6/1 -> Divide_9dd9d/2
  Constant_x_q_cdf13/1 -> Subtract_c46b7/1
  Divide_6307b/1 -> Subtract_def03/1
  Divide_9dd9d/1 -> Subtract_def03/2
  Divide_4ce89/1 -> Blockout_d_psi_gq_SG_D_2_be7cc/1
  Constant_-1_234fe/1 -> Product_dc6e0/1
  State_psi_gq_SG_D_2_a2a06/1 -> Product_dc6e0/2
  Subtract_c46b7/1 -> Product_6d2a7/1
  Subtract_def03/1 -> Product_6d2a7/2
  Product_dc6e0/1 -> Add_1b44c/1
  Add_1b44c/1 -> Divide_4ce89/1
  Constant_T_qd_b549c/1 -> Divide_4ce89/2

== system case2/SG_D_2/d_psi_kq_SG_D_2_block ==
  note: d_psi_kq_SG_D_2 in case2
      | $-\frac{\psi _{\mathrm{gq},\mathrm{SG},D,2}+\psi _{\mathrm{kq},\mathrm{SG},D,2}+\frac{\left(x_{l}-x_{\mathrm{qd}}\right)\,\left(\psi _{q,\mathrm{SG},D,2}+\frac{\psi _{\mathrm{gq},\mathrm{SG},D,2}\,\left(x_{l}-x_{\mathrm{qdd}}\right)}{x_{l}-x_{\mathrm{qd}}}+\frac{\psi _{\mathrm{kq},\mathrm{SG},D,2}\,\left(x_{\mathrm{qd}}-x_{\mathrm{qdd}}\right)}{x_{l}-x_{\mathrm{qd}}}\right)}{x_{\mathrm{qdd}}}}{T_{\mathrm{qdd}}}$
      | Automatically generated on 2025-10-31 18:54:34 .
  State_psi_gq_SG_D_2_2ecc4 : Inport
  State_psi_kq_SG_D_2_ff9b7 : Inport  Port=2
  State_psi_gq_SG_D_2_6238c : Inport  Port=3
  State_psi_kq_SG_D_2_b8096 : Inport  Port=4
  State_psi_q_SG_D_2_76d71 : Inport  Port=5
  Add_30664 : Sum
  Add_3ee67 : Sum
  Add_6d9d5 : Sum
  Add_906fc : Sum
  Add_93a47 : Sum
  Add_ff56f : Sum
  Constant_-1_29f2c : Constant  Value=-1
  Constant_-1_2d5bf : Constant  Value=-1
  Constant_-1_41786 : Constant  Value=-1
  Constant_-1_5a337 : Constant  Value=-1
  Constant_-1_dad9f : Constant  Value=-1
  Constant_T_qdd_28693 : Constant  Value=T_qdd
  Constant_x_l_6d843 : Constant  Value=x_l
  Constant_x_l_a8258 : Constant  Value=x_l
  Constant_x_l_b0aa5 : Constant  Value=x_l
  Constant_x_l_e11d6 : Constant  Value=x_l
  Constant_x_qd_08d80 : Constant  Value=x_qd
  Constant_x_qd_78ece : Constant  Value=x_qd
  Constant_x_qd_a7773 : Constant  Value=x_qd
  Constant_x_qd_e5c17 : Constant  Value=x_qd
  Constant_x_qdd_505b5 : Constant  Value=x_qdd
  Constant_x_qdd_80fae : Constant  Value=x_qdd
  Constant_x_qdd_f8847 : Constant  Value=x_qdd
  Divide_60d66 : Product  Inputs=*/
  Divide_66d7b : Product  Inputs=*/
  Divide_9e2bb : Product  Inputs=*/
  Divide_f33c5 : Product  Inputs=*/
  Product_01a7d : Product
  Product_2b55c : Product
  Product_42c83 : Product
  Product_9456f : Product
  Product_b0cb6 : Product
  Product_d5169 : Product
  Product_e4b6c : Product
  Product_fe210 : Product
  Subtract_643cc : Sum  Inputs=+-
  Subtract_7415e : Sum  Inputs=+-
  Subtract_7e480 : Sum  Inputs=+-
  Blockout_d_psi_kq_SG_D_2_e0637 : Outport
  wires:
  State_psi_kq_SG_D_2_ff9b7/1 -> Subtract_7415e/2
  Constant_-1_29f2c/1 -> Product_e4b6c/1
  Constant_-1_5a337/1 -> Product_fe210/1
  Constant_x_l_b0aa5/1 -> Product_fe210/2
  Constant_x_qdd_f8847/1 -> Add_30664/2
  Constant_x_l_e11d6/1 -> Product_e4b6c/2
  Constant_x_qd_78ece/1 -> Subtract_643cc/1
  Constant_T_qdd_28693/1 -> Divide_f33c5/2
  Constant_-1_2d5bf/1 -> Product_d5169/1
  Product_fe210/1 -> Add_30664/1
  Constant_x_qdd_505b5/1 -> Subtract_643cc/2
  Constant_x_l_a8258/1 -> Product_d5169/2
  Divide_f33c5/1 -> Blockout_d_psi_kq_SG_D_2_e0637/1
  State_psi_gq_SG_D_2_6238c/1 -> Product_42c83/1
  Add_30664/1 -> Product_42c83/2
  Product_e4b6c/1 -> Add_ff56f/1
  Constant_x_qd_08d80/1 -> Add_ff56f/2
  Product_b0cb6/1 -> Divide_60d66/1
  State_psi_kq_SG_D_2_b8096/1 -> Product_9456f/1
  Subtract_643cc/1 -> Product_9456f/2
  Product_d5169/1 -> Add_93a47/1
  Constant_x_qd_e5c17/1 -> Add_93a47/2
  Product_9456f/1 -> Divide_66d7b/1
  Product_42c83/1 -> Divide_9e2bb/1
  Add_ff56f/1 -> Divide_9e2bb/2
  Add_93a47/1 -> Divide_66d7b/2
  State_psi_q_SG_D_2_76d71/1 -> Add_6d9d5/2
  Constant_-1_41786/1 -> Product_01a7d/1
  Constant_x_l_6d843/1 -> Product_01a7d/2
  Divide_9e2bb/1 -> Subtract_7e480/1
  Divide_66d7b/1 -> Subtract_7e480/2
  Product_01a7d/1 -> Add_3ee67/1
  Constant_x_qd_a7773/1 -> Add_3ee67/2
  Subtract_7e480/1 -> Add_6d9d5/1
  Constant_x_qdd_80fae/1 -> Divide_60d66/2
  Constant_-1_dad9f/1 -> Product_2b55c/1
  State_psi_gq_SG_D_2_2ecc4/1 -> Product_2b55c/2
  Add_3ee67/1 -> Product_b0cb6/1
  Add_6d9d5/1 -> Product_b0cb6/2
  Product_2b55c/1 -> Subtract_7415e/1
  Subtract_7415e/1 -> Add_906fc/1
  Divide_60d66/1 -> Add_906fc/2
  Add_906fc/1 -> Divide_f33c5/1

== system case2/SG_D_2/d_psi_q_SG_D_2_block ==
  note: d_psi_q_SG_D_2 in case2
      | $2\,\pi \,f_{0}\,\left(v_{d,\mathrm{SG},D,2}\,\cos\left(\theta _{\mathrm{SG},D,2}\right)+v_{q,\mathrm{SG},D,2}\,\sin\left(\theta _{\mathrm{SG},D,2}\right)-\frac{R_{a}\,\left(\psi _{q,\mathrm{SG},D,2}+\frac{\psi _{\mathrm{gq},\mathrm{SG},D,2}\,\left(x_{l}-x_{\mathrm{qdd}}\right)}{x_{l}-x_{\mathrm{qd}}}+\frac{\psi _{\mathrm{kq},\mathrm{SG},D,2}\,\left(x_{\mathrm{qd}}-x_{\mathrm{qdd}}\right)}{x_{l}-x_{\mathrm{qd}}}\right)}{x_{\mathrm{qdd}}}-\frac{\psi _{d,\mathrm{SG},D,2}\,w_{\mathrm{SG},D,2}}{2\,f_{0}\,\pi }\right)$
      | Automatically generated on 2025-10-31 18:54:16 .
  State_psi_gq_SG_D_2_02402 : Inport
  State_psi_kq_SG_D_2_3ae4e : Inport  Port=2
  State_psi_q_SG_D_2_bc55a : Inport  Port=3
  Input_v_d_SG_D_2_0f316 : Inport  Port=4
  State_theta_SG_D_2_f78f2 : Inport  Port=5
  Input_v_q_SG_D_2_6312d : Inport  Port=6
  State_theta_SG_D_2_25da5 : Inport  Port=7
  State_psi_d_SG_D_2_afeb6 : Inport  Port=8
  State_w_SG_D_2_c2d17 : Inport  Port=9
  Add_038cb : Sum
  Add_66d1f : Sum
  Add_7b870 : Sum
  Add_aa9b4 : Sum
  Add_c22e3 : Sum
  Constant_-1_59267 : Constant  Value=-1
  Constant_-1_a0078 : Constant  Value=-1
  Constant_-1_a0320 : Constant  Value=-1
  Constant_-2.0_c915c : Constant  Value=-2.0
  Constant_2.0_1e6f3 : Constant  Value=2.0
  Constant_R_a_5ca3d : Constant  Value=R_a
  Constant_f0_0be74 : Constant  Value=f0
  Constant_f0_b3d26 : Constant  Value=f0
  Constant_pi_1fd1c : Constant  Value=pi
  Constant_pi_98eb9 : Constant  Value=pi
  Constant_x_l_2e8d2 : Constant  Value=x_l
  Constant_x_l_ad541 : Constant  Value=x_l
  Constant_x_l_c63e7 : Constant  Value=x_l
  Constant_x_qd_9dc82 : Constant  Value=x_qd
  Constant_x_qd_9ee76 : Constant  Value=x_qd
  Constant_x_qd_e88a7 : Constant  Value=x_qd
  Constant_x_qdd_02f1c : Constant  Value=x_qdd
  Constant_x_qdd_4ac45 : Constant  Value=x_qdd
  Constant_x_qdd_4fa83 : Constant  Value=x_qdd
  Divide_0a0be : Product  Inputs=*/
  Divide_c46d6 : Product  Inputs=*/
  Divide_e4fca : Product  Inputs=*/
  Divide_ecf17 : Product  Inputs=*/
  MathFunc_cos_fcd4e : Trigonometry  Operator=cos
  MathFunc_sin_150ee : Trigonometry
  Product_18a59 : Product
  Product_2ccf4 : Product
  Product_2cd09 : Product
  Product_3facd : Product
  Product_500c8 : Product
  Product_71dab : Product
  Product_732da : Product
  Product_b45ac : Product
  Product_c957d : Product
  Product_cde40 : Product
  Product_d6853 : Product
  Product_e6b9c : Product
  Product_e7ccb : Product
  Product_ed51c : Product
  Subtract_13da9 : Sum  Inputs=+-
  Subtract_6a0e8 : Sum  Inputs=+-
  Subtract_8cc31 : Sum  Inputs=+-
  Subtract_b158d : Sum  Inputs=+-
  Blockout_d_psi_q_SG_D_2_71529 : Outport
  wires:
  Constant_x_qdd_02f1c/1 -> Subtract_b158d/2
  Constant_x_l_c63e7/1 -> Product_71dab/2
  Constant_-1_59267/1 -> Product_cde40/1
  Constant_x_l_2e8d2/1 -> Product_cde40/2
  Product_cde40/1 -> Add_7b870/1
  Constant_pi_98eb9/1 -> Product_b45ac/2
  State_psi_gq_SG_D_2_02402/1 -> Product_18a59/1
  Constant_x_l_ad541/1 -> Product_ed51c/2
  State_w_SG_D_2_c2d17/1 -> Product_732da/2
  Constant_x_qd_9ee76/1 -> Add_038cb/2
  Constant_x_qdd_4fa83/1 -> Add_7b870/2
  Constant_2.0_1e6f3/1 -> Product_b45ac/1
  Constant_-1_a0320/1 -> Product_ed51c/1
  Constant_x_qd_e88a7/1 -> Subtract_b158d/1
  Constant_-1_a0078/1 -> Product_71dab/1
  State_psi_q_SG_D_2_bc55a/1 -> Add_c22e3/2
  Add_7b870/1 -> Product_18a59/2
  Product_b45ac/1 -> Product_2ccf4/1
  Product_ed51c/1 -> Add_66d1f/1
  Constant_pi_1fd1c/1 -> Product_c957d/2
  Constant_f0_0be74/1 -> Product_2ccf4/2
  Constant_x_qd_9dc82/1 -> Add_66d1f/2
  State_psi_kq_SG_D_2_3ae4e/1 -> Product_2cd09/1
  Subtract_b158d/1 -> Product_2cd09/2
  Product_71dab/1 -> Add_038cb/1
  Input_v_q_SG_D_2_6312d/1 -> Product_e6b9c/1
  Product_18a59/1 -> Divide_0a0be/1
  Product_2ccf4/1 -> Divide_c46d6/2
  Add_66d1f/1 -> Divide_0a0be/2
  Product_2cd09/1 -> Divide_ecf17/1
  Add_038cb/1 -> Divide_ecf17/2
  Divide_0a0be/1 -> Subtract_6a0e8/1
  State_theta_SG_D_2_f78f2/1 -> MathFunc_cos_fcd4e/1
  Divide_ecf17/1 -> Subtract_6a0e8/2
  Subtract_6a0e8/1 -> Add_c22e3/1
  MathFunc_cos_fcd4e/1 -> Product_e7ccb/2
  Constant_R_a_5ca3d/1 -> Product_500c8/1
  Add_c22e3/1 -> Product_500c8/2
  State_theta_SG_D_2_25da5/1 -> MathFunc_sin_150ee/1
  Product_500c8/1 -> Divide_e4fca/1
  Product_c957d/1 -> Product_3facd/1
  Product_e6b9c/1 -> Subtract_13da9/2
  Constant_x_qdd_4ac45/1 -> Divide_e4fca/2
  Input_v_d_SG_D_2_0f316/1 -> Product_e7ccb/1
  Add_aa9b4/1 -> Product_d6853/2
  Divide_e4fca/1 -> Subtract_8cc31/1
  Product_e7ccb/1 -> Subtract_8cc31/2
  MathFunc_sin_150ee/1 -> Product_e6b9c/2
  Product_d6853/1 -> Blockout_d_psi_q_SG_D_2_71529/1
  State_psi_d_SG_D_2_afeb6/1 -> Product_732da/1
  Constant_-2.0_c915c/1 -> Product_c957d/1
  Product_3facd/1 -> Product_d6853/1
  Subtract_8cc31/1 -> Subtract_13da9/1
  Product_732da/1 -> Divide_c46d6/1
  Constant_f0_b3d26/1 -> Product_3facd/2
  Subtract_13da9/1 -> Add_aa9b4/1
  Divide_c46d6/1 -> Add_aa9b4/2

== system case2/SG_D_2/d_theta_SG_D_2_block ==
  note: d_theta_SG_D_2 in case2
      | $w_{\mathrm{SG},D,2}-2\,\pi \,f_{0}$
      | Automatically generated on 2025-10-31 18:54:41 .
  State_w_SG_D_2_08923 : Inport
  Add_84a88 : Sum
  Constant_-2.0_0921e : Constant  Value=-2.0
  Constant_f0_b7b89 : Constant  Value=f0
  Constant_pi_89bd0 : Constant  Value=pi
  Product_1e552 : Product
  Product_2970b : Product
  Blockout_d_theta_SG_D_2_633fd : Outport
  wires:
  Constant_-2.0_0921e/1 -> Product_1e552/1
  Constant_pi_89bd0/1 -> Product_1e552/2
  Add_84a88/1 -> Blockout_d_theta_SG_D_2_633fd/1
  Product_1e552/1 -> Product_2970b/1
  Constant_f0_b7b89/1 -> Product_2970b/2
  Product_2970b/1 -> Add_84a88/1
  State_w_SG_D_2_08923/1 -> Add_84a88/2
